simulink model "Corneto_flight_program_control"  (R2021a)
settings: Solver=FixedStepAuto  StartTime=0.0  StopTime=inf  RelTol=1e-3
values from neighbouring files (symbols this model uses):
  den_lpf_d = den_lpf20    [Mainframe_init.m]    (also in load_autopilot.m)
  num_lpf_d = num_lpf20    [Mainframe_init.m]    (also in load_autopilot.m)
undefined symbols (not defined in the file or in its folder): Autopilot, AUX, dev, DiscIntNeverNeededParam, Flight_Logic, HIL_Data, Main, pwm_output0, pwm_output1, severity, text, x, y, z
libraries: simulink x22, simulink_extras x20, px4uORBlib x10, px4lib x9, px4Sensorslib x6, dspstat3 x2, sharedtransform x2
(part 1 of 3)
settings Model: ExtModeTrigDuration=10  Creator=sasson  LastModifiedBy=root
settings SolverCC: PositivePriorityOrder=on
settings OptimizationCC: EnhancedBackFolding=on  PassReuseOutputArgsAs=Individual arguments  ZeroExternalMemoryAtStartup=off  ZeroInternalMemoryAtStartup=off  MaxStackSize=64  OptimizeBlockOrder=speed  DifferentSizesBufferReuse=on  OptimizationCustomize=off  EfficientTunableParamExpr=on
settings DebuggingCC: MultiTaskRateTransMsg=warning  ParameterOverflowMsg=none  ParameterTunabilityLossMsg=error
settings HardwareCC: ProdBitPerPointer=32  ProdBitPerSizeT=32  ProdBitPerPtrDiffT=32  ProdLargestAtomicInteger=Long  ProdLargestAtomicFloat=Double  ProdWordSize=32  ProdLongLongMode=on  ProdHWDeviceType=ARM Compatible->ARM Cortex
settings SFSimCC: MATLABDynamicMemAlloc=off  SimTargetLang=C++
settings RTWCC: SystemTargetFile=ert.tlc  HardwareBoard=PX4 Pixhawk 2.1 (Cube)  TLCOptions="-aInlineSetEventsForThisBaseRateFcn=TLC_FALSE -aSuppressMultiTaskScheduler=TLC_FALSE  -aRateBasedStepFcn=0"  TemplateMakefile=ert_default_tmf  Toolchain=GNU Tools for PX4 Autopilots  TargetLang=C++
settings CodeAppCC: ForceParamTrailComments=on  IgnoreCustomStorageClasses=off  OperatorAnnotations=on  SimulinkDataObjDesc=on  SFDataObjDesc=on  InsertBlockDesc=on
settings ERTTargetCC: ExtModeTransport=3  ExtModeStaticAlloc=on  ExtModeStaticAllocSize=1024  ExtModeMexFile=ext_xcp  ExtModeIntrfLevel=Level2 - Open

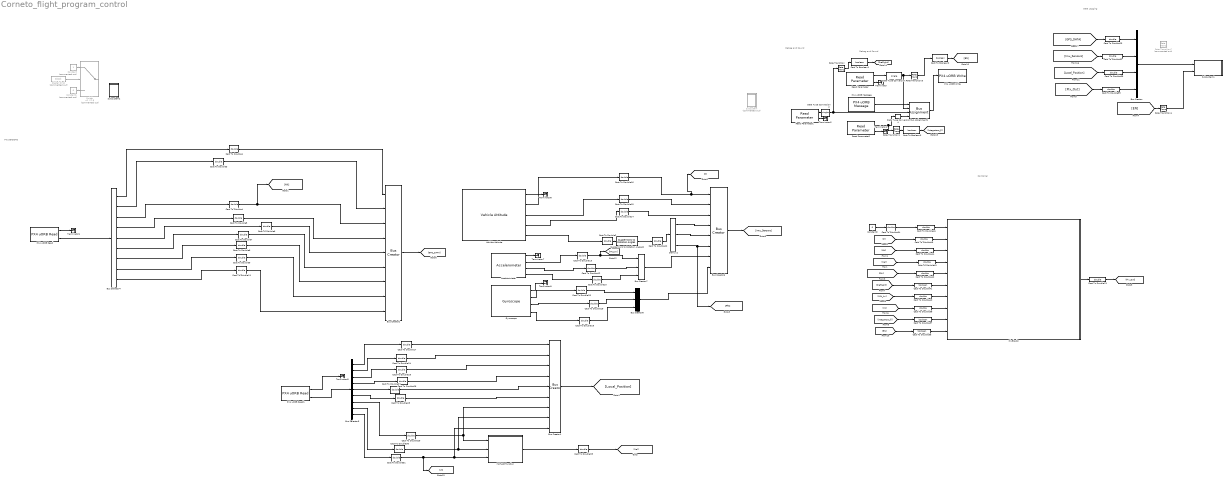
== system Corneto_flight_program_control ==
  note: Debag and Sound
  note: IMU SENSORS
  note: Debag and Sound
  note: Controller
  note: Data Logging
  Accelerometer : px4Sensorslib/Accelerometer  uorbTimeStamp=off  BlockingMode=off  BlockTimeout=1e-3  sampleTime=-1
      settings: SourceProductBaseCode=PX4AUTOPILOTS
  Bus Assignment1 : BusAssignment  AssignedSignals=x,y,z
  Bus Creator1 : BusCreator  Inputs=9
  Bus Creator2 : BusCreator  Inputs=9
  Bus Creator6 : BusCreator  Inputs=8
  Bus Creator7 : BusCreator  Inputs=3
  Bus Creator8 : BusCreator  Inputs=3
  Bus Selector3 : BusSelector  OutputSignals=ax,ay,az,z,x,y,vx,vy,vz
  Bus Selector4 : BusSelector  OutputSignals=lat,lon,alt,fix_type,satellites_used,vel_m_s,vel_n_m_s,vel_e_m_s,vel_d_m_s
  Bus Creator : BusCreator  Inputs=4
  Cast To Boolean1 : DataTypeConversion  OutDataTypeStr=boolean
  Cast To Boolean2 : DataTypeConversion  OutDataTypeStr=boolean
  Cast To Boolean3 : DataTypeConversion  OutDataTypeStr=boolean
  Cast To Double{1..35,38..40,42..46} (43 alike) : DataTypeConversion  OutDataTypeStr=double
  Cast To Double36 : DataTypeConversion  OutDataTypeStr=boolean
  Cast To Double37 : DataTypeConversion  OutDataTypeStr=boolean
  Cast To Double41 : DataTypeConversion  OutDataTypeStr=boolean
  Constant : Constant  Commented=on  OutDataTypeStr=boolean
  Constant1 : Constant  Commented=on  Value=0  OutDataTypeStr=boolean
  Constant2 : Constant  Value=0  SampleTime=-1
  Data Type Conversion2 : DataTypeConversion  OutDataTypeStr=single
  Data Type Conversion3 : DataTypeConversion  OutDataTypeStr=single
  Data Type Conversion4 : DataTypeConversion  OutDataTypeStr=single
  Demux2 : Demux  Outputs=3
  Digital Clock : DigitalClock  Commented=on
  Gyroscope : px4Sensorslib/Gyroscope  uorbTimeStamp=off  BlockingMode=off  BlockTimeout=1e-3  sampleTime=-1
      settings: SourceProductBaseCode=PX4AUTOPILOTS
  MATLAB Function : MATLAB Function  TreatAsAtomicUnit=on
  PX4 uORB Message : px4uORBlib/PX4 uORB Message  uORBTopic=debug_vect  SampleTime=1  selectInstance=debug_vect
      settings: SourceProductBaseCode=PX4AUTOPILOTS
  PX4 uORB Read : px4uORBlib/PX4 uORB Read  uORBTopic=vehicle_gps_position  selectInstance=vehicle_gps_position  SampleTime=-1  BlockingMode=off  BlockTimeout=1e-3
      settings: SourceProductBaseCode=PX4AUTOPILOTS
  PX4 uORB Read1 : px4uORBlib/PX4 uORB Read  uORBTopic=vehicle_local_position  selectInstance=vehicle_local_position  SampleTime=-1  BlockingMode=off  BlockTimeout=1e-3
      settings: SourceProductBaseCode=PX4AUTOPILOTS
  PX4 uORB Write : px4uORBlib/PX4 uORB Write  uORBTopic=debug_vect  selectInstance=debug_vect  MessageQueueLen=1
      settings: SourceProductBaseCode=PX4AUTOPILOTS
  PixBlock2 : Subsystem
  Quaternions to Rotation Angles2 : sharedtransform/Quaternions to Rotation Angles  rotationOrder=ZYX  aMode=aMode
      settings: SourceProductBaseCode=AE,PW,DR,MT,UV,VE
  Rate Transition : RateTransition  InitialCondition=1
  Rate Transition1 : RateTransition  InitialCondition=1
  Rate Transition2 : RateTransition  Commented=on  InitialCondition=0.005  OutPortSampleTime=0.001
  Rate Transition3 : RateTransition  InitialCondition=1
  Rate Transition4 : RateTransition  InitialCondition=0.001  OutPortSampleTime=1
  Read Parameter : px4lib/Read Parameter  ParameterName=SD_save_flag  DataType=INT32  SampleTime=1
      settings: SourceProductBaseCode=PX4AUTOPILOTS
  Read Parameter1 : px4lib/Read Parameter  ParameterName=Preflight_flag  DataType=INT32  SampleTime=1
      settings: SourceProductBaseCode=PX4AUTOPILOTS
  Read Parameter2 : px4lib/Read Parameter  ParameterName=Integrators_flag  DataType=INT32  SampleTime=1
      settings: SourceProductBaseCode=PX4AUTOPILOTS
  Subsystem : Subsystem  Commented=on
  Subsystem1 : Subsystem
  Subsystem2 : Subsystem
  Switch : Switch  Commented=on  Threshold=8
  Terminator{,1..4,7..9} (8 alike) : Terminator
  Vehicle Attitude : px4Sensorslib/Vehicle Attitude  rollRate=on  pitchRate=on  yawRate=on  quaternion=on  uorbTimeStamp=off  BlockingMode=off  BlockTimeout=0.001  sampleTime=-1
      settings: SourceProductBaseCode=PX4AUTOPILOTS
  wires:
  Digital Clock/1 -> Switch/2
  Cast To Double16/1 -> Bus Creator6/1, [P]
  Cast To Boolean1/1 -> [Preflight]
  Constant/1 -> Switch/1
  Cast To Double15/1 -> Bus Creator6/2
  Bus Selector4/7 -> Cast To Double8/1  "<vel_n_m_s>"
  Cast To Double3/1 -> Bus Creator2/2
  Constant1/1 -> Switch/3
  Cast To Double43/1 -> PixBlock2/4(Velocity)
  Rate Transition1/1 -> Cast To Boolean3/1
  Bus Creator2/1 -> [GPS_DATA]
  Cast To Double18/1 -> Bus Creator8/3
  Bus Selector3/5 -> Cast To Double27/1  "<x>"
  Cast To Double40/1 -> PixBlock2/7(IMU_Ax)
  Cast To Double6/1 -> Bus Creator2/5
  Bus Selector3/2 -> Cast To Double24/1  "<ay>"
  Cast To Double1/1 -> Bus Creator2/1
  Bus Selector3/9 -> Cast To Double31/1  "<vz>"
  Rate Transition/1 -> Cast To Boolean1/1
  Rate Transition4/1 -> Subsystem1/2(EN)
  Cast To Double31/1 -> [Vz], Bus Creator1/9, MATLAB Function/3(vz)
  Cast To Double45/1 -> PixBlock2/2(P_rms)
  Read Parameter1/2 -> Terminator2/1
  Bus Creator6/1 -> [Imu_Sensors]
  [Integrators_fl] -> Cast To Double37/1
  [EN] -> Cast To Double36/1
  Cast To Double8/1 -> Bus Creator2/7
  Bus Selector4/4 -> Cast To Double5/1  "<fix_type>"
  PixBlock2/1(Pix_Out) -> Cast To Double21/1
  Vehicle Attitude/3 -> Cast To Double15/1  "q"
  [Local_Position] -> Cast To Double35/1
  Cast To Double5/1 -> Bus Creator2/4
  Cast To Double2/1 -> Quaternions to Rotation Angles2/1
  Bus Selector4/3 -> Cast To Double4/1  "<alt>"
  Cast To Double36/1 -> PixBlock2/10(Integrators1)
  Read Parameter/2 -> Terminator/1
  Cast To Double24/1 -> Bus Creator1/2
  Data Type Conversion3/1 -> Rate Transition3/1, Bus Assignment1/2
  Data Type Conversion4/1 -> Bus Assignment1/4
  Bus Selector3/4 -> Cast To Double26/1  "<z>"
  Accelerometer/3 -> Cast To Double12/1  "accY"
  Cast To Double7/1 -> Bus Creator2/6
  Cast To Double38/1 -> PixBlock2/8(Vz)
  Cast To Double44/1 -> PixBlock2/3(Alt)
  Cast To Double23/1 -> Bus Creator/1
  Cast To Double41/1 -> PixBlock2/6(Preflight)
  Gyroscope/4 -> Cast To Double18/1  "gyroZ"
  Bus Selector4/1 -> Cast To Double1/1  "<lat>"
  Cast To Double46/1 -> PixBlock2/1(Phi_cmd)
  Cast To Double42/1 -> PixBlock2/5(Phi)
  Bus Selector4/9 -> Cast To Double11/1  "<vel_d_m_s>"
  Cast To Double37/1 -> PixBlock2/9(Integrators)
  [Phi] -> Cast To Double42/1
  Demux2/2 -> Bus Creator6/5  "theta"
  Cast To Double12/1 -> Bus Creator7/2
  [Imu_Sensors] -> Cast To Double32/1
  Data Type Conversion2/1 -> Bus Assignment1/3, Rate Transition/1
  [Preflight] -> Cast To Double41/1
  Cast To Double25/1 -> Bus Creator1/3
  [GPS_DATA] -> Cast To Double23/1
  PX4 uORB Read/2 -> Bus Selector4/1
  Cast To Double14/1 -> Bus Creator6/3
  Accelerometer/4 -> Cast To Double10/1  "accZ"
  Bus Selector3/7 -> Cast To Double29/1  "<vx>"
  Vehicle Attitude/2 -> Cast To Double16/1  "p"
  Vehicle Attitude/1 -> Terminator8/1
  [Alt] -> Cast To Double44/1
  Read Parameter2/2 -> Terminator4/1
  Read Parameter/1 -> Data Type Conversion3/1
  [Vz] -> Cast To Double38/1
  Cast To Double13/1 -> [IMU_Ax], Bus Creator7/1
  Bus Selector3/1 -> Cast To Double17/1  "<ax>"
  Read Parameter1/1 -> Data Type Conversion2/1
  Cast To Double4/1 -> Bus Creator2/3, [Alt]
  Read Parameter2/1 -> Rate Transition1/1, Data Type Conversion4/1
  Constant2/1 -> Cast To Double34/1
  [Pix_Out] -> Cast To Double39/1
  [Vel] -> Cast To Double43/1
  Cast To Double22/1 -> Demux2/1
  Bus Selector4/2 -> Cast To Double3/1  "<lon>"
  PX4 uORB Message/1 -> Bus Assignment1/1
  Accelerometer/1 -> Terminator7/1
  Quaternions to Rotation Angles2/1 -> Cast To Double22/1  "euler from PX conj"
  Bus Selector3/8 -> Cast To Double30/1  "<vy>"
  Bus Creator8/1 -> Bus Creator6/8  "gyro"
  Cast To Boolean2/1 -> [EN]
  Cast To Double32/1 -> Bus Creator/2
  Cast To Double19/1 -> Bus Creator8/2
  Cast To Double10/1 -> Bus Creator7/3
  Cast To Double29/1 -> Bus Creator1/7, MATLAB Function/1(vx)
  Cast To Double35/1 -> Bus Creator/3
  Gyroscope/2 -> Cast To Double20/1  "gyroX"
  Bus Selector4/8 -> Cast To Double9/1  "<vel_e_m_s>"
  PX4 uORB Read1/2 -> Bus Selector3/1
  Cast To Double11/1 -> Bus Creator2/9
  Gyroscope/3 -> Cast To Double19/1  "gyroY"
  Bus Selector4/6 -> Cast To Double7/1  "<vel_m_s>"
  [P] -> Cast To Double45/1
  Cast To Double20/1 -> Bus Creator8/1
  PX4 uORB Read/1 -> Terminator1/1
  Cast To Double17/1 -> Bus Creator1/1
  Gyroscope/1 -> Terminator9/1
  Cast To Double27/1 -> Bus Creator1/5
  Bus Selector3/3 -> Cast To Double25/1  "<az>"
  PX4 uORB Read1/1 -> Terminator3/1
  Demux2/1 -> Bus Creator6/4  "psi"
  Cast To Double26/1 -> Bus Creator1/4
  [IMU_Ax] -> Cast To Double40/1
  Cast To Double9/1 -> Bus Creator2/8
  Cast To Double34/1 -> Cast To Double46/1
  Cast To Double39/1 -> Bus Creator/4
  Cast To Double21/1 -> [Pix_Out]
  Bus Assignment1/1 -> PX4 uORB Write/1
  Vehicle Attitude/5 -> Cast To Double2/1
  MATLAB Function/1(y) -> Cast To Double33/1
  Bus Selector4/5 -> Cast To Double6/1  "<satellites_used>"
  Cast To Double28/1 -> Bus Creator1/6
  Cast To Double30/1 -> Bus Creator1/8, MATLAB Function/2(vy)
  Cast To Boolean3/1 -> [Integrators_fl]
  Bus Creator7/1 -> Bus Creator6/7  "accelerometer"
  Bus Selector3/6 -> Cast To Double28/1  "<y>"
  Cast To Double33/1 -> [Vel]
  Accelerometer/2 -> Cast To Double13/1  "accX"
  Bus Creator1/1 -> [Local_Position]
  Vehicle Attitude/4 -> Cast To Double14/1  "r"
  Demux2/3 -> [Phi], Bus Creator6/6  "phi"
  [EN] -> Rate Transition4/1
  Rate Transition3/1 -> Cast To Boolean2/1
  Bus Creator/1 -> Subsystem1/1(Pix_log)

== system Corneto_flight_program_control/PixBlock2 ==
  Phi_cmd : Inport
  P_rms : Inport  Port=2
  Alt : Inport  Port=3
  Velocity : Inport  Port=4
  Phi : Inport  Port=5
  Preflight : Inport  Port=6
  IMU_Ax : Inport  Port=7
  Vz : Inport  Port=8
  Integrators : Inport  Port=9
  Integrators1 : Inport  Port=10
  100 Hz : DiscretePulseGenerator  PulseType=Time based  Period=0.01  PulseWidth=50
  Emulated Pixhawk : Subsystem
  Pix_Out : Outport
  wires:
  100 Hz/1 -> Emulated Pixhawk/Trigger
  Phi_cmd/1 -> Emulated Pixhawk/1(Phi_cmd)
  P_rms/1 -> Emulated Pixhawk/2(P_rms)
  Phi/1 -> Emulated Pixhawk/5(Phi)
  Velocity/1 -> Emulated Pixhawk/4(Velocity)
  Alt/1 -> Emulated Pixhawk/3(Alt)
  IMU_Ax/1 -> Emulated Pixhawk/6(IMU_Ax)
  Vz/1 -> Emulated Pixhawk/7(Vz)
  Preflight/1 -> Emulated Pixhawk/8(Preflight)
  Integrators/1 -> Emulated Pixhawk/9(Integrators)
  Integrators1/1 -> Emulated Pixhawk/10(SD_save_flag)
  Emulated Pixhawk/1(Pix_Out) -> Pix_Out/1

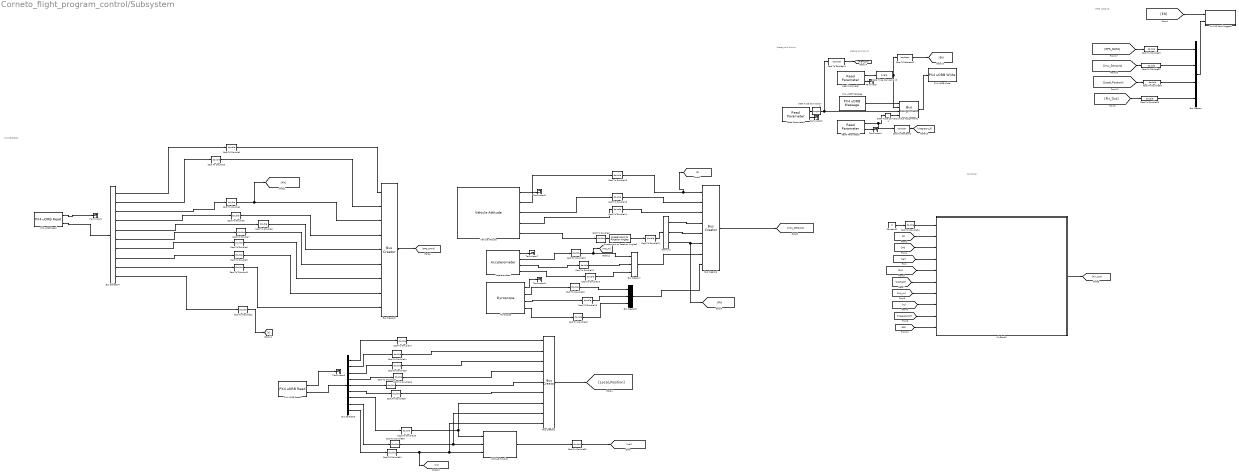
== system Corneto_flight_program_control/Subsystem ==
  note: IMU SENSORS
  note: Debag and Sound
  note: Debag and Sound
  note: Data Logging
  note: Controller
  Accelerometer : px4Sensorslib/Accelerometer  uorbTimeStamp=off  BlockingMode=off  BlockTimeout=1e-3  sampleTime=-1
      settings: SourceProductBaseCode=PX4AUTOPILOTS
  Bus Assignment1 : BusAssignment  AssignedSignals=x,y,z
  Bus Creator1 : BusCreator  Inputs=9
  Bus Creator2 : BusCreator  Inputs=9
  Bus Creator6 : BusCreator  Inputs=8
  Bus Creator7 : BusCreator  Inputs=3
  Bus Creator8 : BusCreator  Inputs=3
  Bus Selector3 : BusSelector  OutputSignals=ax,ay,az,z,x,y,vx,vy,vz
  Bus Selector4 : BusSelector  OutputSignals=lat,lon,alt,fix_type,satellites_used,vel_m_s,vel_n_m_s,vel_e_m_s,vel_d_m_s,timestamp
  Bus Creator : BusCreator  Inputs=4
  Cast To Boolean1 : DataTypeConversion  OutDataTypeStr=boolean
  Cast To Boolean2 : DataTypeConversion  OutDataTypeStr=boolean
  Cast To Boolean3 : DataTypeConversion  OutDataTypeStr=boolean
  Cast To Double{1..35,39} (36 alike) : DataTypeConversion  OutDataTypeStr=double
  Constant2 : Constant  Value=0  SampleTime=-1
  Data Type Conversion2 : DataTypeConversion  OutDataTypeStr=single
  Data Type Conversion3 : DataTypeConversion  OutDataTypeStr=single
  Data Type Conversion4 : DataTypeConversion  OutDataTypeStr=single
  Demux2 : Demux  Outputs=3
  Gyroscope : px4Sensorslib/Gyroscope  uorbTimeStamp=off  BlockingMode=off  BlockTimeout=1e-3  sampleTime=-1
      settings: SourceProductBaseCode=PX4AUTOPILOTS
  MATLAB Function : MATLAB Function  TreatAsAtomicUnit=on
  PX4 SD Card Logger3 : Subsystem  mask(PX4 SD Card Logger){logfile=/fs/microsd/log, logfilename=pwm, cacheflag=off, numRecs=100000000000000}
      mask prompts: logfile "Log Folder"; logfilename "Log File Name"; cacheflag "Cache in Memory"; numRecs "Maximum Record Count"
      mask help:
      | Log data to a specified file on the SD card
      |
      | The block accepts two inputs, enable and data. The incoming data is logged into the SD card when the enable signal is high and the number of data points logged is less than the Maximum Record Count specified.
      |
      | The specified folder should be present in the SD card for logging.
      |
      | If Cache in Memory is unchecked, the data is written to the SD card at every timestep.  If Cache in Memory is checked, data is cached in the memory and is written to SD card only when enable goes low or when the number of data points logged reaches the Maximum Record Count specified.
      mask init:
      | logname=uint8([logfile,'/',logfilename]);
      mask Help: eval('codertarget.internal.helpView(''px4'',''px4sdcardexample'')');
      mask Display:
      | fprintf([get_param(gcb,'logfile'),'/',get_param(gcb,'logfilename')])
      | port_label('input',1,'en')
      | port_label('input',2,'data')
  PX4 uORB Message : px4uORBlib/PX4 uORB Message  uORBTopic=debug_vect  SampleTime=1  selectInstance=debug_vect
      settings: SourceProductBaseCode=PX4AUTOPILOTS
  PX4 uORB Read : px4uORBlib/PX4 uORB Read  uORBTopic=vehicle_gps_position  selectInstance=vehicle_gps_position  SampleTime=-1  BlockingMode=off  BlockTimeout=1e-3
      settings: SourceProductBaseCode=PX4AUTOPILOTS
  PX4 uORB Read1 : px4uORBlib/PX4 uORB Read  uORBTopic=vehicle_local_position  selectInstance=vehicle_local_position  SampleTime=-1  BlockingMode=off  BlockTimeout=1e-3
      settings: SourceProductBaseCode=PX4AUTOPILOTS
  PX4 uORB Write : px4uORBlib/PX4 uORB Write  uORBTopic=debug_vect  selectInstance=debug_vect  MessageQueueLen=1
      settings: SourceProductBaseCode=PX4AUTOPILOTS
  PixBlock2 : Subsystem
  Quaternions to Rotation Angles2 : sharedtransform/Quaternions to Rotation Angles  rotationOrder=ZYX  aMode=aMode
      settings: SourceProductBaseCode=AE,PW,DR,MT,UV,VE
  Read Parameter : px4lib/Read Parameter  ParameterName=SD_save_flag  DataType=INT32  SampleTime=1
      settings: SourceProductBaseCode=PX4AUTOPILOTS
  Read Parameter1 : px4lib/Read Parameter  ParameterName=Preflight_flag  DataType=INT32  SampleTime=1
      settings: SourceProductBaseCode=PX4AUTOPILOTS
  Read Parameter2 : px4lib/Read Parameter  ParameterName=Integrators_flag  DataType=INT32  SampleTime=1
      settings: SourceProductBaseCode=PX4AUTOPILOTS
  Terminator{,1..4,7..9} (8 alike) : Terminator
  Vehicle Attitude : px4Sensorslib/Vehicle Attitude  rollRate=on  pitchRate=on  yawRate=on  quaternion=on  uorbTimeStamp=off  BlockingMode=off  BlockTimeout=0.001  sampleTime=-1
      settings: SourceProductBaseCode=PX4AUTOPILOTS
  wires:
  Vehicle Attitude/3 -> Cast To Double15/1  "q"
  Bus Selector4/6 -> Cast To Double7/1  "<vel_m_s>"
  PX4 uORB Read/2 -> Bus Selector4/1
  Data Type Conversion4/1 -> Bus Assignment1/4
  PX4 uORB Read1/2 -> Bus Selector3/1
  Gyroscope/4 -> Cast To Double18/1  "gyroZ"
  Demux2/1 -> Bus Creator6/4  "psi"
  Bus Creator6/1 -> [Imu_Sensors]
  Bus Selector3/1 -> Cast To Double17/1  "<ax>"
  Cast To Double7/1 -> Bus Creator2/6
  Bus Selector4/9 -> Cast To Double11/1  "<vel_d_m_s>"
  Vehicle Attitude/2 -> Cast To Double16/1  "p"
  Bus Creator2/1 -> [GPS_DATA]
  [Alt] -> PixBlock2/3(Alt)
  Cast To Double34/1 -> PixBlock2/1(Phi_cmd)
  PX4 uORB Read1/1 -> Terminator3/1
  Bus Selector4/3 -> Cast To Double4/1  "<alt>"
  Bus Selector3/9 -> Cast To Double31/1  "<vz>"
  Cast To Double30/1 -> Bus Creator1/8, MATLAB Function/2(vy)
  Demux2/3 -> [Phi], Bus Creator6/6  "phi"
  Vehicle Attitude/4 -> Cast To Double14/1  "r"
  [Integrators_fl] -> PixBlock2/9(Integrators)
  Cast To Double18/1 -> Bus Creator8/3
  Cast To Double33/1 -> [Vel]
  Cast To Double24/1 -> Bus Creator1/2
  Cast To Double16/1 -> Bus Creator6/1, [P]
  Vehicle Attitude/1 -> Terminator8/1
  Bus Selector4/8 -> Cast To Double9/1  "<vel_e_m_s>"
  Cast To Double21/1 -> [A]
  Cast To Double28/1 -> Bus Creator1/6
  Cast To Double8/1 -> Bus Creator2/7
  Bus Creator7/1 -> Bus Creator6/7  "accelerometer"
  Cast To Double17/1 -> Bus Creator1/1
  Bus Selector3/3 -> Cast To Double25/1  "<az>"
  Cast To Double10/1 -> Bus Creator7/3
  Cast To Boolean3/1 -> [Integrators_fl]
  Demux2/2 -> Bus Creator6/5  "theta"
  Bus Selector3/8 -> Cast To Double30/1  "<vy>"
  Bus Creator/1 -> PX4 SD Card Logger3/2(Data)
  Cast To Double11/1 -> Bus Creator2/9
  Vehicle Attitude/5 -> Cast To Double2/1
  Cast To Double9/1 -> Bus Creator2/8
  Cast To Double1/1 -> Bus Creator2/1
  Bus Selector3/4 -> Cast To Double26/1  "<z>"
  [P] -> PixBlock2/2(P_rms)
  Cast To Double29/1 -> Bus Creator1/7, MATLAB Function/1(vx)
  MATLAB Function/1(y) -> Cast To Double33/1
  Cast To Double39/1 -> Bus Creator/4
  Bus Creator1/1 -> [Local_Position]
  Accelerometer/2 -> Cast To Double13/1  "accX"
  Cast To Double25/1 -> Bus Creator1/3
  Cast To Double26/1 -> Bus Creator1/4
  Cast To Boolean1/1 -> [Preflight]
  Bus Selector4/1 -> Cast To Double1/1  "<lat>"
  Accelerometer/4 -> Cast To Double10/1  "accZ"
  Bus Selector3/6 -> Cast To Double28/1  "<y>"
  Cast To Double35/1 -> Bus Creator/3
  Cast To Double4/1 -> Bus Creator2/3, [Alt]
  Bus Selector4/7 -> Cast To Double8/1  "<vel_n_m_s>"
  PX4 uORB Read/1 -> Terminator1/1
  Cast To Double3/1 -> Bus Creator2/2
  Cast To Double14/1 -> Bus Creator6/3
  Cast To Double15/1 -> Bus Creator6/2
  PixBlock2/1(Pix_Out) -> [Pix_Out]
  Data Type Conversion3/1 -> Bus Assignment1/2, Cast To Boolean2/1
  Cast To Double13/1 -> [IMU_Ax], Bus Creator7/1
  Bus Selector3/2 -> Cast To Double24/1  "<ay>"
  Cast To Double19/1 -> Bus Creator8/2
  Bus Selector3/7 -> Cast To Double29/1  "<vx>"
  Gyroscope/3 -> Cast To Double19/1  "gyroY"
  Gyroscope/2 -> Cast To Double20/1  "gyroX"
  Cast To Double20/1 -> Bus Creator8/1
  Read Parameter1/1 -> Data Type Conversion2/1
  Quaternions to Rotation Angles2/1 -> Cast To Double22/1  "euler from PX conj"
  Cast To Double5/1 -> Bus Creator2/4
  Gyroscope/1 -> Terminator9/1
  Cast To Double27/1 -> Bus Creator1/5
  Cast To Double2/1 -> Quaternions to Rotation Angles2/1
  Bus Selector4/4 -> Cast To Double5/1  "<fix_type>"
  Accelerometer/1 -> Terminator7/1
  [Phi] -> PixBlock2/5(Phi)
  Cast To Double6/1 -> Bus Creator2/5
  [Vel] -> PixBlock2/4(Velocity)
  Bus Creator8/1 -> Bus Creator6/8  "gyro"
  Accelerometer/3 -> Cast To Double12/1  "accY"
  Cast To Double12/1 -> Bus Creator7/2
  Bus Selector3/5 -> Cast To Double27/1  "<x>"
  Cast To Double22/1 -> Demux2/1
  Bus Selector4/10 -> Cast To Double21/1  "<timestamp>"
  Cast To Double31/1 -> [Vz], Bus Creator1/9, MATLAB Function/3(vz)
  Read Parameter1/2 -> Terminator2/1
  Bus Selector4/2 -> Cast To Double3/1  "<lon>"
  Constant2/1 -> Cast To Double34/1
  Cast To Double32/1 -> Bus Creator/2
  Bus Selector4/5 -> Cast To Double6/1  "<satellites_used>"
  Cast To Double23/1 -> Bus Creator/1
  PX4 uORB Message/1 -> Bus Assignment1/1
  Bus Assignment1/1 -> PX4 uORB Write/1
  Read Parameter/2 -> Terminator/1
  Cast To Boolean2/1 -> [EN]
  [EN] -> PixBlock2/10(Integrators1)
  [Pix_Out] -> Cast To Double39/1
  [EN] -> PX4 SD Card Logger3/1(En)
  Read Parameter2/1 -> Cast To Boolean3/1, Data Type Conversion4/1
  Read Parameter/1 -> Data Type Conversion3/1
  Data Type Conversion2/1 -> Bus Assignment1/3, Cast To Boolean1/1
  [IMU_Ax] -> PixBlock2/7(IMU_Ax)
  Read Parameter2/2 -> Terminator4/1
  [Preflight] -> PixBlock2/6(Preflight)
  [Vz] -> PixBlock2/8(Vz)
  [Local_Position] -> Cast To Double35/1
  [Imu_Sensors] -> Cast To Double32/1
  [GPS_DATA] -> Cast To Double23/1

== system Corneto_flight_program_control/Subsystem1 ==
  Pix_log : Inport
  EN : Inport  Port=2
  Bus Selector4 : BusSelector  OutputSignals=signal1,signal2,signal3,signal4
  Bus Creator : BusCreator  Inputs=4
  Cast To Double{23,32,35,39} (4 alike) : DataTypeConversion  OutDataTypeStr=double
  PX4 SD Card Logger3 : Subsystem  mask(PX4 SD Card Logger){logfile=/fs/microsd/log, logfilename=pwm, cacheflag=off, numRecs=100000000000000}
      mask prompts: logfile "Log Folder"; logfilename "Log File Name"; cacheflag "Cache in Memory"; numRecs "Maximum Record Count"
      mask help:
      | Log data to a specified file on the SD card
      |
      | The block accepts two inputs, enable and data. The incoming data is logged into the SD card when the enable signal is high and the number of data points logged is less than the Maximum Record Count specified.
      |
      | The specified folder should be present in the SD card for logging.
      |
      | If Cache in Memory is unchecked, the data is written to the SD card at every timestep.  If Cache in Memory is checked, data is cached in the memory and is written to SD card only when enable goes low or when the number of data points logged reaches the Maximum Record Count specified.
      mask init:
      | logname=uint8([logfile,'/',logfilename]);
      mask Help: eval('codertarget.internal.helpView(''px4'',''px4sdcardexample'')');
      mask Display:
      | fprintf([get_param(gcb,'logfile'),'/',get_param(gcb,'logfilename')])
      | port_label('input',1,'en')
      | port_label('input',2,'data')
  wires:
  Bus Selector4/4 -> Cast To Double39/1  "<signal4>"
  Cast To Double35/1 -> Bus Creator/3
  Bus Selector4/3 -> Cast To Double35/1  "<signal3>"
  Cast To Double32/1 -> Bus Creator/2
  Cast To Double23/1 -> Bus Creator/1
  Bus Selector4/2 -> Cast To Double32/1  "<signal2>"
  Cast To Double39/1 -> Bus Creator/4
  Bus Selector4/1 -> Cast To Double23/1  "<signal1>"
  Pix_log/1 -> Bus Selector4/1
  Bus Creator/1 -> PX4 SD Card Logger3/2(Data)
  EN/1 -> PX4 SD Card Logger3/1(En)

== system Corneto_flight_program_control/Subsystem2 ==
  Bus Assignment : BusAssignment  AssignedSignals=severity,text
  Constant : Constant  Value=7  OutDataTypeStr=uint8
  PX4 uORB Message1 : px4uORBlib/PX4 uORB Message  uORBTopic=mavlink_log  SampleTime=-1  selectInstance=mavlink_log
      settings: SourceProductBaseCode=PX4AUTOPILOTS
  PX4 uORB Write1 : px4uORBlib/PX4 uORB Write  uORBTopic=mavlink_log  selectInstance=mavlink_log  MessageQueueLen=1
      settings: SourceProductBaseCode=PX4AUTOPILOTS
  String Constant : StringConstant  String="\"The fucking Missile is READY! (Hope so)\""
  String to ASCII : StringToASCII  OutputVectorSize=50
  wires:
  String to ASCII/1 -> Bus Assignment/3
  PX4 uORB Message1/1 -> Bus Assignment/1
  String Constant/1 -> String to ASCII/1
  Constant/1 -> Bus Assignment/2
  Bus Assignment/1 -> PX4 uORB Write1/1

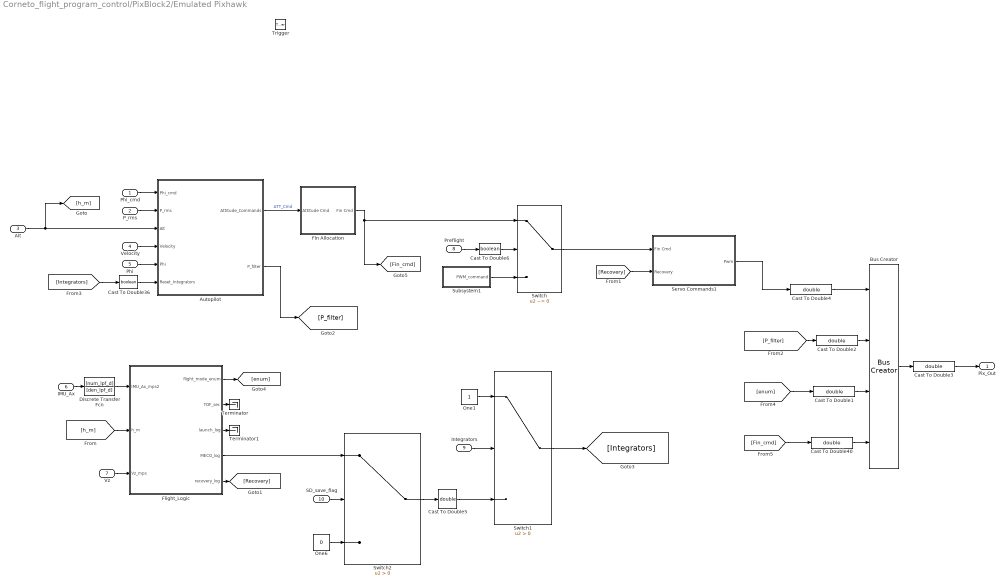
== system Corneto_flight_program_control/PixBlock2/Emulated Pixhawk ==
  Phi_cmd : Inport
  P_rms : Inport  Port=2
  Alt : Inport  Port=3
  Velocity : Inport  Port=4
  Phi : Inport  Port=5
  IMU_Ax : Inport  Port=6
  Vz : Inport  Port=7
  Preflight : Inport  Port=8
  Integrators : Inport  Port=9
  SD_save_flag : Inport  Port=10
  Trigger : TriggerPort  VariantControl=Variant  PortDimensions=1
  Autopilot : Subsystem
  Bus Creator : BusCreator  Inputs=4
  Cast To Double{1..5,40} (6 alike) : DataTypeConversion  OutDataTypeStr=double
  Cast To Double36 : DataTypeConversion  OutDataTypeStr=boolean
  Cast To Double6 : DataTypeConversion  OutDataTypeStr=boolean
  Discrete Transfer Fcn : DiscreteTransferFcn  Numerator=[num_lpf_d]  Denominator=[den_lpf_d]
  Fin Allocation : Subsystem
  Flight_Logic : Subsystem
  One1 : Constant  OutDataTypeStr=Inherit: Inherit via back propagation
  One6 : Constant  Value=0  OutDataTypeStr=Inherit: Inherit via back propagation
  Servo Commands1 : Subsystem
  Subsystem1 : Subsystem
  Switch : Switch  Criteria=u2 ~= 0
  Switch1 : Switch  Criteria=u2 > Threshold
  Switch2 : Switch  Criteria=u2 > Threshold
  Terminator : Terminator
  Terminator1 : Terminator
  Pix_Out : Outport
  wires:
  Alt/1 -> [h_m], Autopilot/3(Alt)
  Autopilot/1(Attitude_Commands) -> Fin Allocation/1(Attitude Cmd)  "ATT_Cmd"
  Phi_cmd/1 -> Autopilot/1(Phi_cmd)
  Velocity/1 -> Autopilot/4(Velocity)
  Phi/1 -> Autopilot/5(Phi)
  P_rms/1 -> Autopilot/2(P_rms)
  Autopilot/2(P_filter) -> [P_filter]
  [Integrators] -> Cast To Double36/1
  IMU_Ax/1 -> Discrete Transfer Fcn/1
  [h_m] -> Flight_Logic/2(h_m)
  Vz/1 -> Flight_Logic/3(Vz_mps)
  Discrete Transfer Fcn/1 -> Flight_Logic/1(IMU_Ax_mps2)
  Flight_Logic/5(recovery_log) -> [Recovery]
  [Recovery] -> Servo Commands1/2(Recovery)
  Flight_Logic/1(flight_mode_enum) -> [enum]
  Flight_Logic/2(TOF_sec) -> Terminator/1
  Flight_Logic/3(launch_log) -> Terminator1/1
  Subsystem1/1(PWM_command) -> Switch/3
  Fin Allocation/1(Fin Cmd) -> Switch/1, [Fin_cmd]
  Servo Commands1/1(Pwm) -> Cast To Double4/1
  Switch/1 -> Servo Commands1/1(Fin Cmd)
  Switch2/1 -> Cast To Double5/1
  Integrators/1 -> Switch1/2
  SD_save_flag/1 -> Switch2/2
  Flight_Logic/4(MECO_log) -> Switch2/1
  One6/1 -> Switch2/3
  One1/1 -> Switch1/1
  Switch1/1 -> [Integrators]
  [P_filter] -> Cast To Double2/1
  Bus Creator/1 -> Cast To Double3/1
  [enum] -> Cast To Double1/1
  [Fin_cmd] -> Cast To Double40/1
  Cast To Double40/1 -> Bus Creator/4
  Cast To Double1/1 -> Bus Creator/3
  Cast To Double2/1 -> Bus Creator/2
  Cast To Double3/1 -> Pix_Out/1
  Cast To Double4/1 -> Bus Creator/1
  Cast To Double5/1 -> Switch1/3
  Cast To Double36/1 -> Autopilot/6(Reset_Integrators)
  Preflight/1 -> Cast To Double6/1
  Cast To Double6/1 -> Switch/2

== system Corneto_flight_program_control/Subsystem/PX4 SD Card Logger3 ==
  En : Inport
  Data : Inport  Port=2
  SDCard_logger : MATLAB Function  TreatAsAtomicUnit=on
  Signal Specification : SignalSpecification  OutDataTypeStr=boolean
  wires:
  Data/1 -> SDCard_logger/2(data)
  En/1 -> Signal Specification/1
  Signal Specification/1 -> SDCard_logger/1(en)

== system Corneto_flight_program_control/Subsystem/PixBlock2 ==
  Phi_cmd : Inport
  P_rms : Inport  Port=2
  Alt : Inport  Port=3
  Velocity : Inport  Port=4
  Phi : Inport  Port=5
  Preflight : Inport  Port=6
  IMU_Ax : Inport  Port=7
  Vz : Inport  Port=8
  Integrators : Inport  Port=9
  Integrators1 : Inport  Port=10
  100 Hz : DiscretePulseGenerator  PulseType=Time based  Period=0.01  PulseWidth=50
  Bus Creator : BusCreator  Inputs=4
  Emulated Pixhawk : Subsystem
  Pix_Out : Outport
  wires:
  100 Hz/1 -> Emulated Pixhawk/Trigger
  Phi_cmd/1 -> Emulated Pixhawk/1(Phi_cmd)
  P_rms/1 -> Emulated Pixhawk/2(P_rms)
  Phi/1 -> Emulated Pixhawk/5(Phi)
  Velocity/1 -> Emulated Pixhawk/4(Velocity)
  Alt/1 -> Emulated Pixhawk/3(Alt)
  IMU_Ax/1 -> Emulated Pixhawk/6(IMU_Ax)
  Vz/1 -> Emulated Pixhawk/7(Vz)
  Preflight/1 -> Emulated Pixhawk/8(Preflight)
  Integrators/1 -> Emulated Pixhawk/9(Integrators)
  Emulated Pixhawk/1(P_filter) -> Bus Creator/1
  Emulated Pixhawk/2(Fin_cms) -> Bus Creator/2
  Emulated Pixhawk/3(PWM) -> Bus Creator/3
  Emulated Pixhawk/4(enum) -> Bus Creator/4
  Integrators1/1 -> Emulated Pixhawk/10(SD_save_flag)
  Bus Creator/1 -> Pix_Out/1

== system Corneto_flight_program_control/Subsystem1/PX4 SD Card Logger3 ==
  En : Inport
  Data : Inport  Port=2
  SDCard_logger : MATLAB Function  TreatAsAtomicUnit=on
  Signal Specification : SignalSpecification  OutDataTypeStr=boolean
  wires:
  Data/1 -> SDCard_logger/2(data)
  En/1 -> Signal Specification/1
  Signal Specification/1 -> SDCard_logger/1(en)

== system Corneto_flight_program_control/PixBlock2/Emulated Pixhawk/Autopilot ==
  Phi_cmd : Inport
  P_rms : Inport  Port=2
  Alt : Inport  Port=3
  Velocity : Inport  Port=4
  Phi : Inport  Port=5
  Reset_Integrators : Inport  Port=6
  Bus Creator3 : BusCreator  Inputs=3
  Discrete Transfer Fcn : DiscreteTransferFcn  Numerator=[num_lpf_d]  Denominator=[den_lpf_d]
  Phi_Control : Subsystem
  Zero : Constant  Value=0  OutDataTypeStr=Inherit: Inherit via back propagation
  Attitude_Commands : Outport  VectorParamsAs1DForOutWhenUnconnected=off
  P_filter : Outport  Port=2  VectorParamsAs1DForOutWhenUnconnected=off
  wires:
  P_rms/1 -> Discrete Transfer Fcn/1
  Velocity/1 -> Phi_Control/5(V_mps)
  Zero/1 -> [Delta_Cmd_Psi], [Delta_Cmd_Theta]
  [Delta_Cmd_Phi] -> Bus Creator3/1  "Phi_Cmd_rad"
  [Delta_Cmd_Theta] -> Bus Creator3/2  "Theta_Cmd_rad"
  Bus Creator3/1 -> Attitude_Commands/1
  [Delta_Cmd_Psi] -> Bus Creator3/3  "Psi_Cmd_rad"
  Alt/1 -> Phi_Control/6(h_m)
  Phi_Control/1(dela_cmd_rad) -> [Delta_Cmd_Phi]  "Phi_Cmd_rad"
  Discrete Transfer Fcn/1 -> P_filter/1, Phi_Control/3(p_rps)
  Phi/1 -> Phi_Control/2(phi_rad)
  Phi_cmd/1 -> Phi_Control/1(phi_cmd_rad)
  Reset_Integrators/1 -> Phi_Control/4(Reset Integrators)

== system Corneto_flight_program_control/PixBlock2/Emulated Pixhawk/Fin Allocation ==
  Attitude Cmd : Inport
  Bus Creator : BusCreator  Inputs=4
  Bus Selector : BusSelector  OutputSignals=Phi_Cmd_rad,Theta_Cmd_rad,Psi_Cmd_rad
  Demux : Demux
  Vector Concatenate1 : Concatenate  NumInputs=3
  control_allocation : Subsystem
  Fin Cmd : Outport  VectorParamsAs1DForOutWhenUnconnected=off
  wires:
  Demux/4 -> Bus Creator/4  "Fin_4_Cmd_rad"
  control_allocation/1(siB_cmd) -> Demux/1
  Bus Selector/3 -> Vector Concatenate1/3  "<Psi_Cmd_rad>"
  Vector Concatenate1/1 -> control_allocation/1(fin_cmd)  "fin_cmd"
  Bus Selector/1 -> Vector Concatenate1/1  "<Phi_Cmd_rad>"
  Demux/3 -> Bus Creator/3  "Fin_3_Cmd_rad"
  Bus Selector/2 -> Vector Concatenate1/2  "<Theta_Cmd_rad>"
  Demux/1 -> Bus Creator/1  "Fin_1_Cmd_rad"
  Bus Creator/1 -> Fin Cmd/1
  Attitude Cmd/1 -> Bus Selector/1
  Demux/2 -> Bus Creator/2  "Fin_2_Cmd_rad"

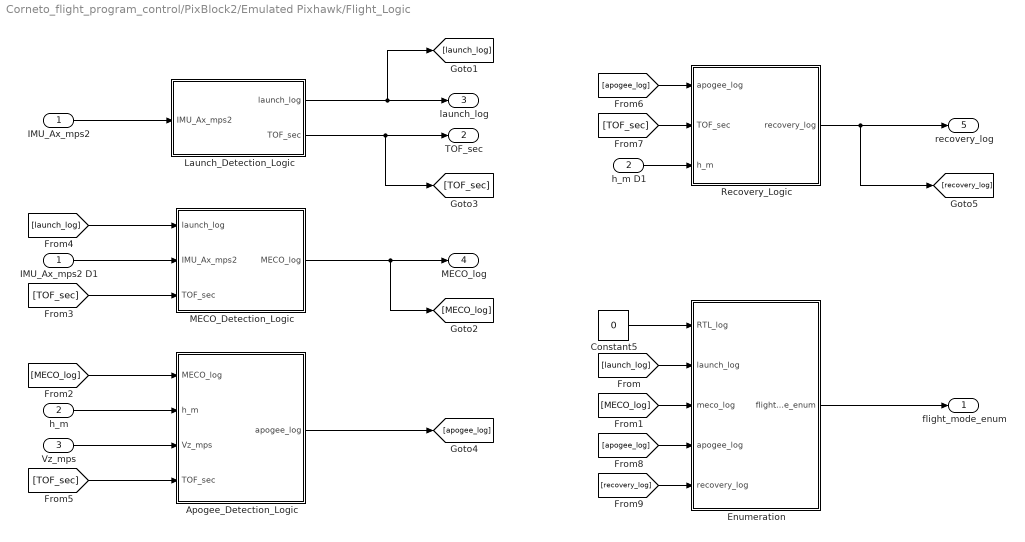
== system Corneto_flight_program_control/PixBlock2/Emulated Pixhawk/Flight_Logic ==
  IMU_Ax_mps2 : Inport
  h_m : Inport  Port=2
  Vz_mps : Inport  Port=3
  Apogee_Detection_Logic : Subsystem
  Constant5 : Constant  Value=0
  Enumeration : Subsystem
  IMU_Ax_mps2 D1 : InportShadow
  Launch_Detection_Logic : Subsystem
  MECO_Detection_Logic : Subsystem
  Recovery_Logic : Subsystem
  h_m D1 : InportShadow  Port=2
  flight_mode_enum : Outport
  TOF_sec : Outport  Port=2
  launch_log : Outport  Port=3
  MECO_log : Outport  Port=4
  recovery_log : Outport  Port=5
  wires:
  Enumeration/1(flight_mode_enum) -> flight_mode_enum/1
  [launch_log] -> Enumeration/2(launch_log)
  [MECO_log] -> Enumeration/3(meco_log)
  IMU_Ax_mps2/1 -> Launch_Detection_Logic/1(IMU_Ax_mps2)
  IMU_Ax_mps2 D1/1 -> MECO_Detection_Logic/2(IMU_Ax_mps2)
  Launch_Detection_Logic/1(launch_log) -> [launch_log], launch_log/1
  Launch_Detection_Logic/2(TOF_sec) -> [TOF_sec], TOF_sec/1
  [launch_log] -> MECO_Detection_Logic/1(launch_log)
  MECO_Detection_Logic/1(MECO_log) -> [MECO_log], MECO_log/1
  [MECO_log] -> Apogee_Detection_Logic/1(MECO_log)
  h_m/1 -> Apogee_Detection_Logic/2(h_m)
  Vz_mps/1 -> Apogee_Detection_Logic/3(Vz_mps)
  Apogee_Detection_Logic/1(apogee_log) -> [apogee_log]
  [TOF_sec] -> MECO_Detection_Logic/3(TOF_sec)
  [TOF_sec] -> Apogee_Detection_Logic/4(TOF_sec)
  Constant5/1 -> Enumeration/1(RTL_log)
  [apogee_log] -> Recovery_Logic/1(apogee_log)
  [TOF_sec] -> Recovery_Logic/2(TOF_sec)
  h_m D1/1 -> Recovery_Logic/3(h_m)
  Recovery_Logic/1(recovery_log) -> [recovery_log], recovery_log/1
  [apogee_log] -> Enumeration/4(apogee_log)
  [recovery_log] -> Enumeration/5(recovery_log)

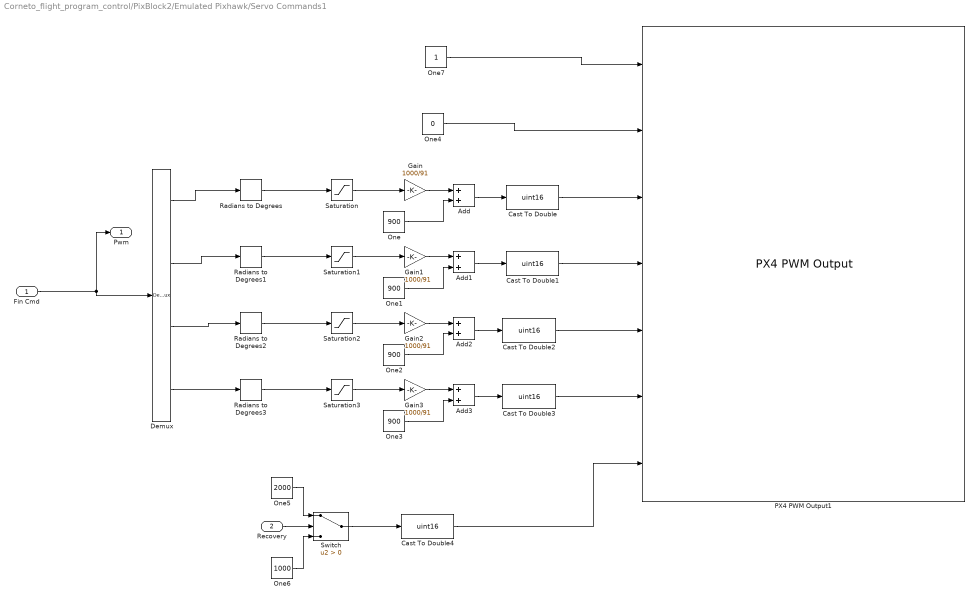
== system Corneto_flight_program_control/PixBlock2/Emulated Pixhawk/Servo Commands1 ==
  Fin Cmd : Inport
  Recovery : Inport  Port=2
  Add{,1..3} (4 alike) : Sum
  Cast To Double{,1..4} (5 alike) : DataTypeConversion  OutDataTypeStr=uint16
  Demux : Demux
  Gain{,1..3} (4 alike) : Gain  Gain=1000/91
  One{,1..3} (4 alike) : Constant  Value=900  OutDataTypeStr=Inherit: Inherit via back propagation
  One4 : Constant  Value=0  OutDataTypeStr=boolean
  One5 : Constant  Value=2000  OutDataTypeStr=Inherit: Inherit via back propagation
  One6 : Constant  Value=1000  OutDataTypeStr=Inherit: Inherit via back propagation
  One7 : Constant  OutDataTypeStr=boolean
  PX4 PWM Output1 : px4lib/PX4 PWM Output  pwmDevice=Main (/dev/pwm_output0)  pwmChannel1_=on  pwmChannel2_=on  pwmChannel3_=on  pwmChannel4_=on  pwmChannel5_=on  pwmChannel6_=off  pwmChannel7_=off  pwmChannel8_=off  forceTerminateFailsafe=off  outputErrorStatus=off
      settings: SourceProductBaseCode=PX4AUTOPILOTS
  Radians to Degrees{,1..3} (4 alike) : simulink_extras/Transformations/Radians to Degrees
  Saturation{,1..3} (4 alike) : Saturate  UpperLimit=20  LowerLimit=-20
  Switch : Switch  Criteria=u2 > Threshold
  Pwm : Outport
  wires:
  One4/1 -> PX4 PWM Output1/2
  Cast To Double4/1 -> PX4 PWM Output1/7
  Recovery/1 -> Switch/2
  One5/1 -> Switch/1
  One6/1 -> Switch/3
  Switch/1 -> Cast To Double4/1
  One7/1 -> PX4 PWM Output1/1
  Fin Cmd/1 -> Demux/1, Pwm/1
  Demux/2 -> Radians to Degrees1/1
  Radians to Degrees2/1 -> Saturation2/1
  Demux/3 -> Radians to Degrees2/1
  Add1/1 -> Cast To Double1/1
  One3/1 -> Add3/2
  Radians to Degrees/1 -> Saturation/1
  Add/1 -> Cast To Double/1
  Saturation/1 -> Gain/1
  One1/1 -> Add1/2
  Demux/4 -> Radians to Degrees3/1
  Add2/1 -> Cast To Double2/1
  One/1 -> Add/2
  Saturation1/1 -> Gain1/1
  Gain3/1 -> Add3/1
  Cast To Double1/1 -> PX4 PWM Output1/4
  Cast To Double3/1 -> PX4 PWM Output1/6
  Radians to Degrees3/1 -> Saturation3/1
  Radians to Degrees1/1 -> Saturation1/1
  Gain1/1 -> Add1/1
  Cast To Double2/1 -> PX4 PWM Output1/5
  Demux/1 -> Radians to Degrees/1
  Gain/1 -> Add/1
  Cast To Double/1 -> PX4 PWM Output1/3
  Add3/1 -> Cast To Double3/1
  Saturation2/1 -> Gain2/1
  Saturation3/1 -> Gain3/1
  Gain2/1 -> Add2/1
  One2/1 -> Add2/2

== system Corneto_flight_program_control/PixBlock2/Emulated Pixhawk/Subsystem1 ==
  Bus Creator : BusCreator  Inputs=4
  Cast To Double{1..3,6} (4 alike) : DataTypeConversion  OutDataTypeStr=double
  Degrees to Radians{,1..3} (4 alike) : simulink_extras/Transformations/Degrees to Radians
  One{5..8} (4 alike) : Constant  Value=5  OutDataTypeStr=Inherit: Inherit via back propagation  SampleTime=-1
  PWM_command : Outport
  wires:
  One5/1 -> Cast To Double6/1  "Fin_1_Cmd_rad"
  One8/1 -> Cast To Double3/1  "Fin_4_Cmd_rad"
  One6/1 -> Cast To Double1/1  "Fin_2_Cmd_rad"
  One7/1 -> Cast To Double2/1  "Fin_3_Cmd_rad"
  Degrees to Radians/1 -> Bus Creator/1
  Degrees to Radians1/1 -> Bus Creator/2
  Degrees to Radians2/1 -> Bus Creator/3
  Degrees to Radians3/1 -> Bus Creator/4
  Bus Creator/1 -> PWM_command/1
  Cast To Double3/1 -> Degrees to Radians3/1
  Cast To Double2/1 -> Degrees to Radians2/1
  Cast To Double1/1 -> Degrees to Radians1/1
  Cast To Double6/1 -> Degrees to Radians/1

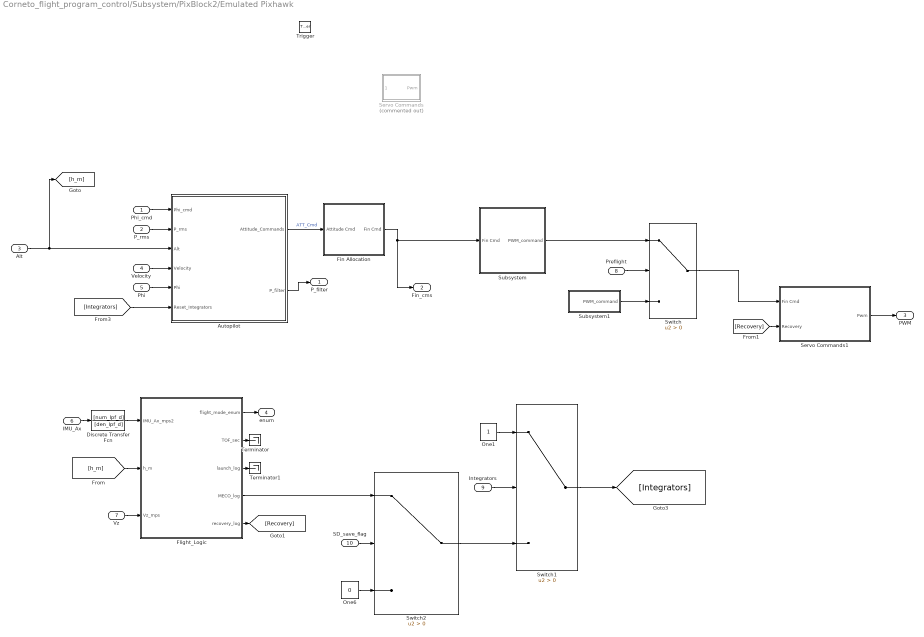
== system Corneto_flight_program_control/Subsystem/PixBlock2/Emulated Pixhawk ==
  Phi_cmd : Inport
  P_rms : Inport  Port=2
  Alt : Inport  Port=3
  Velocity : Inport  Port=4
  Phi : Inport  Port=5
  IMU_Ax : Inport  Port=6
  Vz : Inport  Port=7
  Preflight : Inport  Port=8
  Integrators : Inport  Port=9
  SD_save_flag : Inport  Port=10
  Trigger : TriggerPort  VariantControl=Variant  PortDimensions=1
  Autopilot : Subsystem
  Discrete Transfer Fcn : DiscreteTransferFcn  Numerator=[num_lpf_d]  Denominator=[den_lpf_d]
  Fin Allocation : Subsystem
  Flight_Logic : Subsystem
  One1 : Constant  OutDataTypeStr=Inherit: Inherit via back propagation
  One6 : Constant  Value=0  OutDataTypeStr=Inherit: Inherit via back propagation
  Servo Commands : Subsystem  Commented=on
  Servo Commands1 : Subsystem
  Subsystem : Subsystem
  Subsystem1 : Subsystem
  Switch : Switch  Criteria=u2 > Threshold
  Switch1 : Switch  Criteria=u2 > Threshold
  Switch2 : Switch  Criteria=u2 > Threshold
  Terminator : Terminator
  Terminator1 : Terminator
  P_filter : Outport  VectorParamsAs1DForOutWhenUnconnected=off
  Fin_cms : Outport  Port=2  VectorParamsAs1DForOutWhenUnconnected=off
  PWM : Outport  Port=3  VectorParamsAs1DForOutWhenUnconnected=off
  enum : Outport  Port=4  VectorParamsAs1DForOutWhenUnconnected=off
  wires:
  Alt/1 -> [h_m], Autopilot/3(Alt)
  Autopilot/1(Attitude_Commands) -> Fin Allocation/1(Attitude Cmd)  "ATT_Cmd"
  Phi_cmd/1 -> Autopilot/1(Phi_cmd)
  Velocity/1 -> Autopilot/4(Velocity)
  Phi/1 -> Autopilot/5(Phi)
  P_rms/1 -> Autopilot/2(P_rms)
  Autopilot/2(P_filter) -> P_filter/1
  [Integrators] -> Autopilot/6(Reset_Integrators)
  IMU_Ax/1 -> Discrete Transfer Fcn/1
  [h_m] -> Flight_Logic/2(h_m)
  Vz/1 -> Flight_Logic/3(Vz_mps)
  Discrete Transfer Fcn/1 -> Flight_Logic/1(IMU_Ax_mps2)
  Flight_Logic/5(recovery_log) -> [Recovery]
  [Recovery] -> Servo Commands1/2(Recovery)
  Flight_Logic/1(flight_mode_enum) -> enum/1
  Flight_Logic/2(TOF_sec) -> Terminator/1
  Flight_Logic/3(launch_log) -> Terminator1/1
  Fin Allocation/1(Fin Cmd) -> Fin_cms/1, Subsystem/1(Fin Cmd)
  Subsystem1/1(PWM_command) -> Switch/3
  Subsystem/1(PWM_command) -> Switch/1
  Servo Commands1/1(Pwm) -> PWM/1
  Switch/1 -> Servo Commands1/1(Fin Cmd)
  Preflight/1 -> Switch/2
  Switch2/1 -> Switch1/3
  Integrators/1 -> Switch1/2
  SD_save_flag/1 -> Switch2/2
  Flight_Logic/4(MECO_log) -> Switch2/1
  One6/1 -> Switch2/3
  One1/1 -> Switch1/1
  Switch1/1 -> [Integrators]

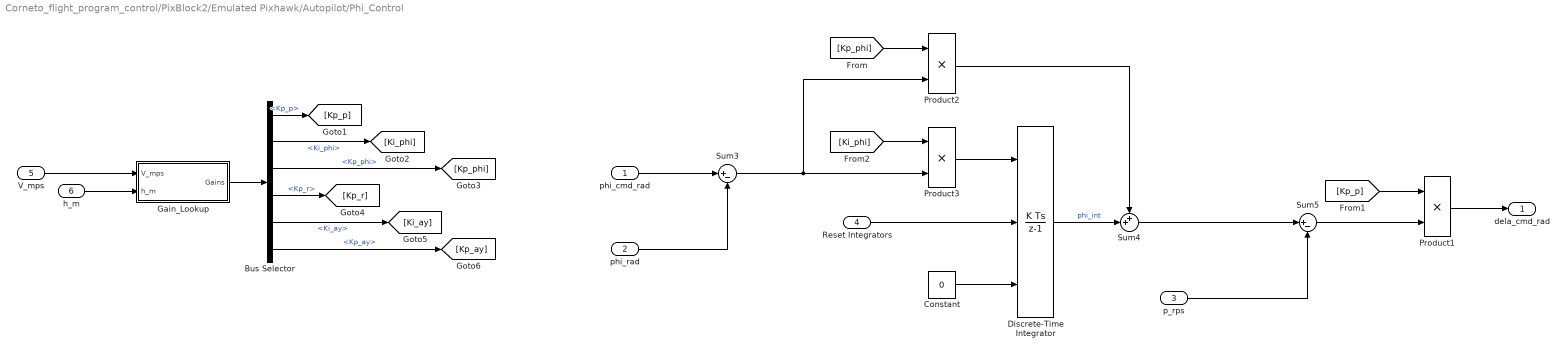
== system Corneto_flight_program_control/PixBlock2/Emulated Pixhawk/Autopilot/Phi_Control ==
  phi_cmd_rad : Inport
  phi_rad : Inport  Port=2
  p_rps : Inport  Port=3
  Reset Integrators : Inport  Port=4
  V_mps : Inport  Port=5
  h_m : Inport  Port=6
  Bus Selector : BusSelector  OutputSignals=Kp_p,Ki_phi,Kp_phi,Kp_r,Ki_ay,Kp_ay
  Constant : Constant  Value=0  OutDataTypeStr=single  SampleTime=-1
  Discrete-Time Integrator : DiscreteIntegrator  ExternalReset=level  InitialConditionSource=external  SampleTime=-1  OutDataTypeStr=single  ICPrevOutput=DiscIntNeverNeededParam  ICPrevScaledInput=DiscIntNeverNeededParam
  Gain_Lookup : Subsystem
  Product1 : Product
  Product2 : Product
  Product3 : Product
  Sum3 : Sum  Inputs=|+-
  Sum4 : Sum  Inputs=++|
  Sum5 : Sum  Inputs=|+-
  dela_cmd_rad : Outport
  wires:
  phi_cmd_rad/1 -> Sum3/1
  Reset Integrators/1 -> Discrete-Time Integrator/2
  p_rps/1 -> Sum5/2
  phi_rad/1 -> Sum3/2
  Product2/1 -> Sum4/1
  Sum3/1 -> Product3/2, Product2/2
  Constant/1 -> Discrete-Time Integrator/3
  Sum5/1 -> Product1/2
  [Ki_phi] -> Product3/1
  Product1/1 -> dela_cmd_rad/1
  [Kp_p] -> Product1/1
  [Kp_phi] -> Product2/1
  Discrete-Time Integrator/1 -> Sum4/2  "phi_int"
  Sum4/1 -> Sum5/1
  Product3/1 -> Discrete-Time Integrator/1
  h_m/1 -> Gain_Lookup/2(h_m)
  Bus Selector/6 -> [Kp_ay]  "<Kp_ay>"
  Bus Selector/5 -> [Ki_ay]  "<Ki_ay>"
  Bus Selector/2 -> [Ki_phi]  "<Ki_phi>"
  Bus Selector/1 -> [Kp_p]  "<Kp_p>"
  V_mps/1 -> Gain_Lookup/1(V_mps)
  Bus Selector/4 -> [Kp_r]  "<Kp_r>"
  Gain_Lookup/1(Gains) -> Bus Selector/1
  Bus Selector/3 -> [Kp_phi]  "<Kp_phi>"

== system Corneto_flight_program_control/PixBlock2/Emulated Pixhawk/Fin Allocation/control_allocation ==
  fin_cmd : Inport
  Constant7 : Constant  Value=HIL_Data.FDM.Tr4r3  OutDataTypeStr=single
  Product : Product  Multiplication=Matrix(*)
  siB_cmd : Outport  VectorParamsAs1DForOutWhenUnconnected=off
  wires:
  Constant7/1 -> Product/1
  fin_cmd/1 -> Product/2
  Product/1 -> siB_cmd/1  "siB_cmd"

== system Corneto_flight_program_control/PixBlock2/Emulated Pixhawk/Flight_Logic/Apogee_Detection_Logic ==
  MECO_log : Inport
  h_m : Inport  Port=2
  Vz_mps : Inport  Port=3
  TOF_sec : Inport  Port=4
  AND : Logic  Inputs=3  AllPortsSameDT=off  OutDataTypeStr=boolean
  AND1 : Logic  Operator=OR  AllPortsSameDT=off  OutDataTypeStr=boolean
  Compare To Constant : simulink/Logic and Bit Operations/Compare To Constant  relop=>  const=0  OutDataTypeStr=boolean
  Compare To Constant1 : simulink/Logic and Bit Operations/Compare To Constant  relop=>=  const=Flight_Logic.h_apogee_timer_threshold_sec  OutDataTypeStr=boolean
      settings: AttributesFormatString=|
      | %<relop>
      | %<const>
  Compare To Constant3 : simulink/Logic and Bit Operations/Compare To Constant  relop=>=  const=Flight_Logic.apogee_timeout_TOF_sec  OutDataTypeStr=boolean
      settings: AttributesFormatString=|
      | %<relop>
      | %<const>
  Detect Decrease : simulink/Logic and Bit Operations/Detect Decrease  vinit=0.0  OutDataTypeStr=uint8
  Enable_Timer_Logic : Subsystem
  Latch_Signal : Subsystem
  Moving Average1 : dspstat3/Moving Average  Method=Sliding window  ForgettingFactorPort=off  SpecifyWindowLength=on  WindowLength=guidc_n_window  ForgettingFactor=0.9  SimulateUsing=Code generation
  apogee_log : Outport
  wires:
  AND1/1 -> apogee_log/1  "apogee_log"
  AND/1 -> Latch_Signal/1(signal)
  h_m/1 -> Moving Average1/1
  MECO_log/1 -> AND/1
  Moving Average1/1 -> Detect Decrease/1  "hBE_mf"
  Detect Decrease/1 -> Enable_Timer_Logic/1(enable_timer)  "flag_I_hBE"
  Enable_Timer_Logic/1(timer) -> Compare To Constant1/1
  Compare To Constant1/1 -> AND/2  "apogee_timer_log"
  Vz_mps/1 -> Compare To Constant/1
  Compare To Constant/1 -> AND/3  "apogee_vz_log"
  Latch_Signal/1(signal_latched) -> AND1/1  "apogee_latched"
  TOF_sec/1 -> Compare To Constant3/1
  Compare To Constant3/1 -> AND1/2  "apogee_timeout_log"

== system Corneto_flight_program_control/PixBlock2/Emulated Pixhawk/Flight_Logic/Enumeration ==
  RTL_log : Inport
  launch_log : Inport  Port=2
  meco_log : Inport  Port=3
  apogee_log : Inport  Port=4
  recovery_log : Inport  Port=5
  Constant : Constant
  Constant1 : Constant  Value=200
  Constant2 : Constant  Value=300
  Constant3 : Constant  Value=400
  Constant4 : Constant  Value=600
  Constant5 : Constant  Value=0
  Constant6 : Constant  Value=500
  Switch{,1..4} (5 alike) : Switch  Criteria=u2 ~= 0
  Terminator : Terminator
  flight_mode_enum : Outport
  wires:
  Switch/1 -> Switch1/3
  Constant3/1 -> Switch2/1
  Constant4/1 -> Switch3/1
  RTL_log/1 -> Switch/2
  Constant1/1 -> Switch/1
  Constant/1 -> Switch/3
  Switch3/1 -> flight_mode_enum/1  "flight_mode_enum"
  meco_log/1 -> Switch2/2
  launch_log/1 -> Switch1/2
  Constant2/1 -> Switch1/1
  Switch2/1 -> Switch4/3
  Switch1/1 -> Switch2/3
  Constant5/1 -> Switch4/2
  Constant6/1 -> Switch4/1
  Switch4/1 -> Switch3/3
  recovery_log/1 -> Switch3/2
  apogee_log/1 -> Terminator/1

== system Corneto_flight_program_control/PixBlock2/Emulated Pixhawk/Flight_Logic/Launch_Detection_Logic ==
  IMU_Ax_mps2 : Inport
  AND : Logic  AllPortsSameDT=off  OutDataTypeStr=boolean
  Compare To Constant : simulink/Logic and Bit Operations/Compare To Constant  relop=>=  const=Flight_Logic.Ax_launch_accel_threshold_mps2  OutDataTypeStr=boolean
      settings: AttributesFormatString=|
      | %<relop>
      | %<const>
  Compare To Constant1 : simulink/Logic and Bit Operations/Compare To Constant  relop=>=  const=Flight_Logic.Ax_launch_timer_threshold_sec  OutDataTypeStr=boolean
      settings: AttributesFormatString=|
      | %<relop>
      | %<const>
  Constant : Constant  Value=0
  Enable_Timer_Logic : Subsystem
  Latch_Signal : Subsystem
  Memory : Memory  InheritSampleTime=on  LinearizeAsDelay=on
  Switch : Switch  Criteria=u2 ~= 0
  launch_log : Outport
  TOF_sec : Outport  Port=2
  wires:
  Compare To Constant/1 -> AND/1, Enable_Timer_Logic/1(accel_threshold_log)  "launch_Ax_log"
  Enable_Timer_Logic/1(time_since_launch) -> Switch/1, Compare To Constant1/1
  Compare To Constant1/1 -> AND/2  "launch_timer_log"
  AND/1 -> Latch_Signal/1(signal)
  IMU_Ax_mps2/1 -> Compare To Constant/1
  Latch_Signal/1(signal_latched) -> [launch_latched], launch_log/1  "launch_log"
  [launch_latched] -> Memory/1
  Memory/1 -> Enable_Timer_Logic/2(launch_latched)
  [launch_latched] -> Switch/2
  Switch/1 -> TOF_sec/1  "TOF_sec"
  Constant/1 -> Switch/3

== system Corneto_flight_program_control/PixBlock2/Emulated Pixhawk/Flight_Logic/MECO_Detection_Logic ==
  launch_log : Inport
  IMU_Ax_mps2 : Inport  Port=2
  TOF_sec : Inport  Port=3
  AND : Logic  AllPortsSameDT=off  OutDataTypeStr=boolean
  AND1 : Logic  Operator=OR  AllPortsSameDT=off  OutDataTypeStr=boolean
  Compare To Constant1 : simulink/Logic and Bit Operations/Compare To Constant  relop=>=  const=Flight_Logic.Ax_MECO_timer_threshold_sec  OutDataTypeStr=boolean
      settings: AttributesFormatString=|
      | %<relop>
      | %<const>
  Compare To Constant2 : simulink/Logic and Bit Operations/Compare To Constant  relop=<=  const=0  OutDataTypeStr=boolean
      settings: AttributesFormatString=|
      | %<relop>
      | %<const>
  Compare To Constant3 : simulink/Logic and Bit Operations/Compare To Constant  relop=>=  const=Flight_Logic.MECO_timeout_TOF_sec  OutDataTypeStr=boolean
      settings: AttributesFormatString=|
      | %<relop>
      | %<const>
  Enable_Timer_Logic : Subsystem
  Latch_Signal : Subsystem
  MECO_log : Outport
  wires:
  launch_log/1 -> AND/1
  IMU_Ax_mps2/1 -> Compare To Constant2/1
  Enable_Timer_Logic/1(timer) -> Compare To Constant1/1
  Compare To Constant1/1 -> Latch_Signal/1(signal)  "MECO_timer_log"
  AND/1 -> Enable_Timer_Logic/1(enable_timer)
  AND1/1 -> MECO_log/1  "MECO_log"
  Compare To Constant2/1 -> AND/2  "MECO_Ax_log"
  Latch_Signal/1(signal_latched) -> AND1/1  "MECO_latched"
  TOF_sec/1 -> Compare To Constant3/1
  Compare To Constant3/1 -> AND1/2  "MECO_timeout_log"

== system Corneto_flight_program_control/PixBlock2/Emulated Pixhawk/Flight_Logic/Recovery_Logic ==
  apogee_log : Inport
  TOF_sec : Inport  Port=2
  h_m : Inport  Port=3
  AND1 : Logic  Operator=OR  AllPortsSameDT=off  OutDataTypeStr=boolean
  AND2 : Logic  AllPortsSameDT=off  OutDataTypeStr=boolean
  Compare To Constant1 : simulink/Logic and Bit Operations/Compare To Constant  relop=>=  const=Flight_Logic.apogee_recovery_timer_threshold_sec  OutDataTypeStr=boolean
      settings: AttributesFormatString=|
      | %<relop>
      | %<const>
  Compare To Constant3 : simulink/Logic and Bit Operations/Compare To Constant  relop=>=  const=Flight_Logic.recovery_timeout_TOF_sec  OutDataTypeStr=boolean
      settings: AttributesFormatString=|
      | %<relop>
      | %<const>
  Constant : Constant  Value=Flight_Logic.disable_recovery_manual
      settings: AttributesFormatString=%<Value>
  Enable_Timer_Logic : Subsystem
  Latch_Signal : Subsystem
  NOT : Logic  Operator=NOT  AllPortsSameDT=off  OutDataTypeStr=boolean
  Terminator : Terminator
  recovery_log : Outport
  wires:
  Compare To Constant3/1 -> AND1/2  "recovery_timeout_log"
  TOF_sec/1 -> Compare To Constant3/1
  Latch_Signal/1(signal_latched) -> AND1/1  "recovery_latched"
  AND1/1 -> AND2/1
  apogee_log/1 -> Enable_Timer_Logic/1(enable_timer)
  Compare To Constant1/1 -> Latch_Signal/1(signal)  "apogee_recovery_timer_log"
  Enable_Timer_Logic/1(timer) -> Compare To Constant1/1
  h_m/1 -> Terminator/1
  AND2/1 -> recovery_log/1  "recovery_log"
  Constant/1 -> NOT/1  "disable_recovery_manual"
  NOT/1 -> AND2/2
